simulink model "Htest2"  (R2014a)
settings: Solver=ode45  StartTime=0.0  StopTime=0.1  RelTol=1e-3
libraries: sh_lib x13, fl_lib x10, nesl_utility x10
settings Model: SimulationMode=accelerator  Creator=Zhenyu  LastModifiedBy=Zhenyu

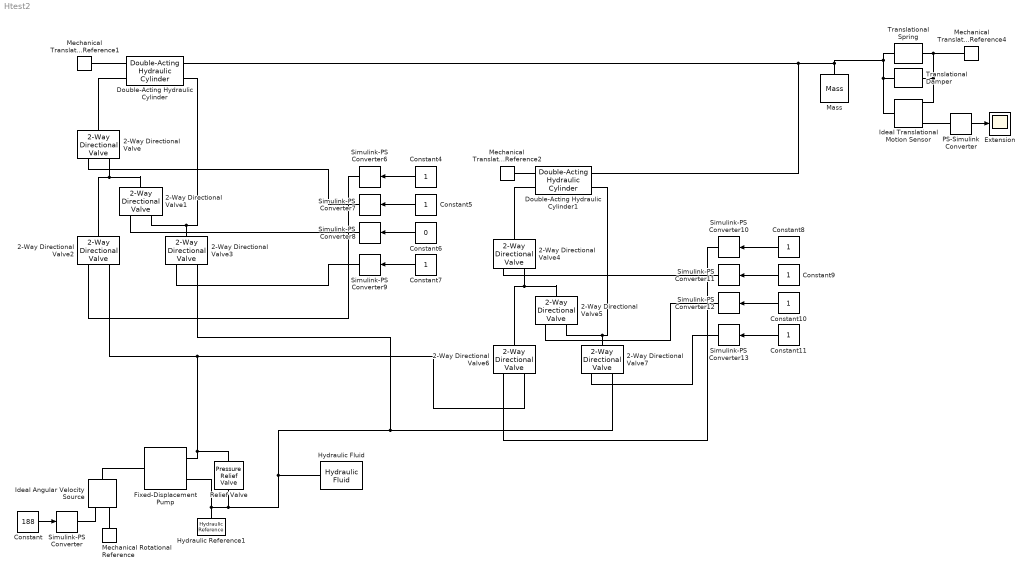
== system Htest2 ==
  2-Way Directional Valve{,1..7} (8 alike) : sh_lib/Valves/Directional Valves/2-Way Directional Valve  mdl_type=1  area_max=5e-5 m^2  opening_max=0.005 m  opening_tab=[ -0.002 0 0.002 0.005 0.015 ] m  area_tab=[ 1e-9 2.0352e-7 4.0736e-5 1.1438e-4 3.4356e-4 ] m^2  pressure_tab=[ -1e+7 -5e+6 -2e+6 2e+6 5e+6 1e+7 ] Pa  flow_rate_tab=[ -1e-7 -7.0711e-8 -4.4721e-8 4.4721e-8 7.0711e-8 1e-7; -2.0352e-5 -1.4391e-5 -9.1017e-6 9.1017e-6 1.4391e-5 2.0352e-5; -0.0040736 -0.0028805 -0.0018218 0.0018218 0.0028805 0.0040736; -0.011438 -0.0080879 -0.0051152 0.0051152 0.0080879 0.011438; -0.034356 -0.024293 -0.015364 0.015364 0.024293 0.034356 ] m^3/s  interp_method=1  extrap_method=1  C_d=0.7  x_0=0 m  Re_cr=12  A_leak=1e-12 m^2
  Constant : Constant  Value=188
  Constant{4..5,7..11} (7 alike) : Constant
  Constant6 : Constant  Value=0
  Double-Acting Hydraulic Cylinder : sh_lib/Hydraulic Cylinders/Double-Acting Hydraulic Cylinder  area_A=1e-3 m^2  area_B=0.5e-3 m^2  stroke=0.2 m  init_pos=0 m  dead_vol_A=1e-4 m^3  dead_vol_B=1e-4 m^3  init_pressure_A=0 Pa  init_pressure_B=0 Pa  k_sh=1.4  stiff=1e6 N/m  D=150 N/(m/s)  or=1  or_sign=1
  Double-Acting Hydraulic Cylinder1 : sh_lib/Hydraulic Cylinders/Double-Acting Hydraulic Cylinder  area_A=2e-3 m^2  area_B=1e-3 m^2  stroke=0.2 m  init_pos=0 m  dead_vol_A=1e-4 m^3  dead_vol_B=1e-4 m^3  init_pressure_A=0 Pa  init_pressure_B=0 Pa  k_sh=1.4  stiff=1e6 N/m  D=150 N/(m/s)  or=1  or_sign=1
  Extension : Scope
      settings: TimeRange=10  YMin=-0.2  YMax=0.6000000000000001  SaveName=Actuation_System_DATA
  Fixed-Displacement Pump : sh_lib/Pumps and Motors/Fixed-Displacement Pump  D=5e-04 m^3/rad  efficiency_vol=0.92  efficiency_tot=0.8  pr_nominal=1e+7 Pa  w_nominal=188 rad/s  visc_nominal=18 cSt  dens_nominal=900 kg/m^3  k_leak=1e-11 m^3/s/Pa  efficiency_mech=0.7
  Hydraulic Reference1 : fl_lib/Hydraulic/Hydraulic Elements/Hydraulic Reference
  Hydraulic Fluid : sh_lib/Hydraulic Utilities/Hydraulic Fluid  DataSource=1  SelFluid=24  SysTemp=60 c  TrapAir=0.005  ViscDerFactor=1  range_error=2
  Ideal Angular Velocity Source : fl_lib/Mechanical/Mechanical Sources/Ideal Angular Velocity Source
  Ideal Translational Motion Sensor : fl_lib/Mechanical/Mechanical Sensors/Ideal Translational Motion Sensor  offset=0 m
  Mass : fl_lib/Mechanical/Translational Elements/Mass  mass=10 kg  v_specify=on  v_priority=High  v=0 m/s  f_specify=off  f_priority=High  f=0 N
  Mechanical Rotational Reference : fl_lib/Mechanical/Rotational Elements/Mechanical Rotational Reference
  Mechanical Translational Reference1 : fl_lib/Mechanical/Translational Elements/Mechanical Translational Reference  Tag=Factory Generic
  Mechanical Translational Reference2 : fl_lib/Mechanical/Translational Elements/Mechanical Translational Reference  Tag=Factory Generic
  Mechanical Translational Reference4 : fl_lib/Mechanical/Translational Elements/Mechanical Translational Reference  Tag=Factory Generic
  PS-Simulink Converter : nesl_utility/PS-Simulink Converter  PhysicalDomain=network_engine_domain  SubClassName=ps_output  LeftPortType=input  RightPortType=output  PseudoPeriodic=off  Frequencies=[]  Unit=1  AffineConversion=off
  Relief Valve : sh_lib/Valves/Pressure Control Valves/Pressure Relief Valve  area_max=2e-4 m^2  pres_set=3e7 Pa  reg_range=3e6 Pa  C_d=0.7  Re_cr=12  A_leak=1e-12 m^2  gain=1 m^2/Pa  pr_max=55e5 Pa
  Simulink-PS Converter : nesl_utility/Simulink-PS Converter  PhysicalDomain=network_engine_domain  SubClassName=ps_input  LeftPortType=input  RightPortType=output  PseudoPeriodic=off  Frequencies=[]  NoiseDistribution=none  NoiseParameters=[]  Unit=rad/s  AffineConversion=off  InputFiltering=off  SimscapeFilterOrder=1  InputFilterTimeConstant=.001  UdotUserProvided=0
  Simulink-PS Converter{6..13} (8 alike) : nesl_utility/Simulink-PS Converter  PhysicalDomain=network_engine_domain  SubClassName=ps_input  LeftPortType=input  RightPortType=output  PseudoPeriodic=off  Frequencies=[]  NoiseDistribution=none  NoiseParameters=[]  Unit=m  AffineConversion=off  InputFiltering=off  SimscapeFilterOrder=1  InputFilterTimeConstant=.001  UdotUserProvided=1
  Translational Damper : fl_lib/Mechanical/Translational Elements/Translational Damper  D=100 N/(m/s)  v_specify=off  v_priority=High  v=0 m/s  f_specify=off  f_priority=High  f=0 N
  Translational Spring : fl_lib/Mechanical/Translational Elements/Translational Spring  spr_rate=1000 N/m  v_specify=off  v_priority=High  v=0 m/s  f_specify=off  f_priority=High  f=0 N  x_specify=on  x_priority=High  x=0 m
  wires:
  Constant4/1 -> Simulink-PS Converter6/1
  Constant5/1 -> Simulink-PS Converter7/1
  Constant6/1 -> Simulink-PS Converter8/1
  Constant7/1 -> Simulink-PS Converter9/1
  Constant8/1 -> Simulink-PS Converter10/1
  Constant9/1 -> Simulink-PS Converter11/1
  Constant10/1 -> Simulink-PS Converter12/1
  Constant11/1 -> Simulink-PS Converter13/1
  Constant/1 -> Simulink-PS Converter/1
  PS-Simulink Converter/1 -> Extension/1
  connections:
  Double-Acting Hydraulic Cylinder/LConn1 -- Mechanical Translational Reference1/LConn1
  Double-Acting Hydraulic Cylinder1/LConn1 -- Mechanical Translational Reference2/LConn1
  2-Way Directional Valve2/RConn1 -- 2-Way Directional Valve1/RConn1 -- 2-Way Directional Valve/LConn2
  2-Way Directional Valve3/RConn1 -- Double-Acting Hydraulic Cylinder/RConn2 -- 2-Way Directional Valve1/LConn2
  2-Way Directional Valve/RConn1 -- Double-Acting Hydraulic Cylinder/LConn2
  2-Way Directional Valve4/LConn2 -- 2-Way Directional Valve6/RConn1 -- 2-Way Directional Valve5/RConn1
  2-Way Directional Valve5/LConn2 -- Double-Acting Hydraulic Cylinder1/RConn2 -- 2-Way Directional Valve7/RConn1
  Double-Acting Hydraulic Cylinder1/LConn2 -- 2-Way Directional Valve4/RConn1
  Mass/LConn1 -- Translational Spring/LConn1 -- Ideal Translational Motion Sensor/LConn1 -- Translational Damper/LConn1 -- Double-Acting Hydraulic Cylinder1/RConn1 -- Double-Acting Hydraulic Cylinder/RConn1
  Relief Valve/RConn1 -- 2-Way Directional Valve7/LConn2 -- 2-Way Directional Valve3/LConn2 -- Hydraulic Fluid/RConn1 -- Hydraulic Reference1/LConn1 -- Fixed-Displacement Pump/RConn2
  Fixed-Displacement Pump/RConn1 -- 2-Way Directional Valve6/LConn2 -- 2-Way Directional Valve2/LConn2 -- Relief Valve/LConn1
  Simulink-PS Converter10/RConn1 -- 2-Way Directional Valve6/LConn1
  Simulink-PS Converter11/RConn1 -- 2-Way Directional Valve4/LConn1
  Simulink-PS Converter12/RConn1 -- 2-Way Directional Valve5/LConn1
  Simulink-PS Converter13/RConn1 -- 2-Way Directional Valve7/LConn1
  Simulink-PS Converter6/RConn1 -- 2-Way Directional Valve2/LConn1
  Simulink-PS Converter7/RConn1 -- 2-Way Directional Valve/LConn1
  Simulink-PS Converter8/RConn1 -- 2-Way Directional Valve1/LConn1
  Simulink-PS Converter9/RConn1 -- 2-Way Directional Valve3/LConn1
  Mechanical Rotational Reference/LConn1 -- Ideal Angular Velocity Source/RConn2
  Simulink-PS Converter/RConn1 -- Ideal Angular Velocity Source/RConn1
  Ideal Angular Velocity Source/LConn1 -- Fixed-Displacement Pump/LConn1
  Translational Spring/RConn1 -- Mechanical Translational Reference4/LConn1 -- Translational Damper/RConn1 -- Ideal Translational Motion Sensor/RConn1
  PS-Simulink Converter/LConn1 -- Ideal Translational Motion Sensor/RConn3
